simulink model "angle_model"  (R2016b)
settings: Solver=VariableStepAuto  StartTime=0.0  StopTime=10.0  RelTol=1e-3
undefined symbols (not defined in the file): magnitude
settings Model: Creator=202008840  LastModifiedBy=202008840

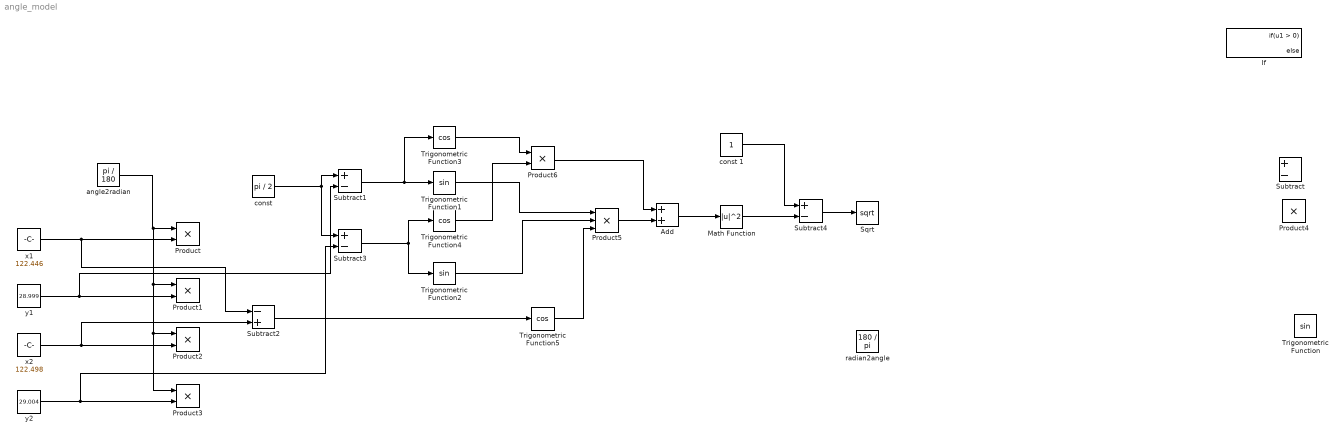
== system angle_model ==
  Add : Sum
  If : If  NumInputs=2
  Math Function : Math  Operator=magnitude^2  SaturateOnIntegerOverflow=on
  Product{,1..4,6} (6 alike) : Product
  Product5 : Product  Inputs=3
  Sqrt : Sqrt  SaturateOnIntegerOverflow=on
  Subtract{,1,3..4} (4 alike) : Sum  Inputs=+-
  Subtract2 : Sum  Inputs=-+
  Trigonometric Function : Trigonometry
  Trigonometric Function1 : Trigonometry
  Trigonometric Function2 : Trigonometry
  Trigonometric Function3 : Trigonometry  Operator=cos
  Trigonometric Function4 : Trigonometry  Operator=cos
  Trigonometric Function5 : Trigonometry  Operator=cos
  angle2radian : Constant  Value=pi / 180
  const : Constant  Value=pi / 2
  const 1 : Constant
  radian2angle : Constant  Value=180 / pi
  x1 : Constant  Value=122.446
  x2 : Constant  Value=122.498
  y1 : Constant  Value=28.999
  y2 : Constant  Value=29.004
  wires:
  x1/1 -> Subtract2/1, Product/2
  y1/1 -> Subtract1/2, Product1/2
  x2/1 -> Subtract2/2, Product2/2
  y2/1 -> Subtract3/2, Product3/2
  angle2radian/1 -> Product3/1, Product2/1, Product1/1, Product/1
  const/1 -> Subtract1/1, Subtract3/1
  Subtract2/1 -> Trigonometric Function5/1
  Subtract1/1 -> Trigonometric Function3/1, Trigonometric Function1/1
  Subtract3/1 -> Trigonometric Function4/1, Trigonometric Function2/1
  Trigonometric Function1/1 -> Product5/1
  Trigonometric Function2/1 -> Product5/2
  Trigonometric Function3/1 -> Product6/1
  Trigonometric Function4/1 -> Product6/2
  Trigonometric Function5/1 -> Product5/3
  Product6/1 -> Add/1
  Product5/1 -> Add/2
  const 1/1 -> Subtract4/1
  Subtract4/1 -> Sqrt/1
  Add/1 -> Math Function/1
  Math Function/1 -> Subtract4/2
